simulink model "SHIP_DOWN_matlab_2017"  (R2018b)
settings: Solver=ode8  StartTime=0.0  StopTime=1  RelTol=1e-3
undefined symbols (not defined in the file): Cout_c, Cout_r, Cvh_c, Cvh_r, dellay_f1, dellay_f2, dellay_f3, dellay_f4, dellay_f5, dellay_f6, DiscIntNeverNeededParam, f, L1_l, L1_r, R_out, Uout, Uvh, Uvh_r
libraries: powerlib x40, simulink x7, simulink_extras x6, dspstat3 x4, powerlib_meascontrol x2
settings Model: Creator=Anton  LastModifiedBy=VID Company
settings SFSimCC: SimUseLocalCustomCode=off
settings RTWCC: RTWUseLocalCustomCode=off
settings CodeAppCC: StateflowObjectComments=on
settings SimscapeCC: SimscapeNormalizeSystem=off

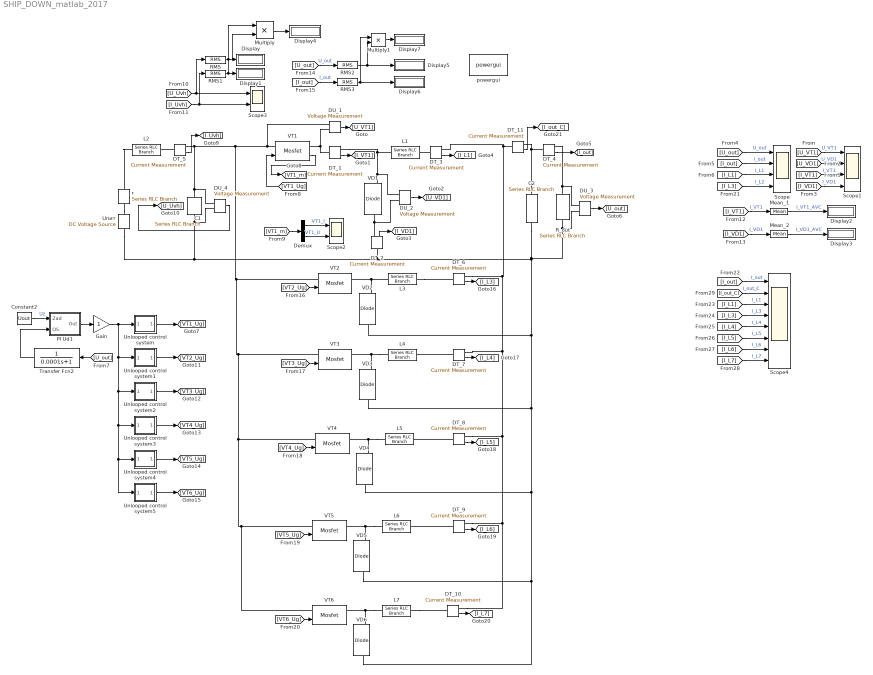
== system SHIP_DOWN_matlab_2017 ==
  C1 : powerlib/Elements/Series RLC Branch  LConnTagsString=__new0  RConnTagsString=__new0  BranchType=RC  Resistance=Cvh_r  Inductance=1e-3  SetiL0=off  InitialCurrent=0  Capacitance=Cvh_c  Setx0=on  InitialVoltage=Uvh  Measurements=Branch voltage
      settings: SourceProductName=Simscape Electrical
  C2 : powerlib/Elements/Series RLC Branch  LConnTagsString=__new0  RConnTagsString=__new0  BranchType=RC  Resistance=Cout_r  Inductance=1e-3  SetiL0=off  InitialCurrent=0  Capacitance=Cout_c  Setx0=on  InitialVoltage=Uout  Measurements=Branch voltage
      settings: SourceProductName=Simscape Electrical
  Constant2 : Constant  Value=Uout
  DT_{1..11} (11 alike) : powerlib/Measurements/Current Measurement  PhasorSimulation=off  OutputType=Complex  PSBequivalent=0
      settings: SourceProductName=Simscape Electrical
  DU_{1..4} (4 alike) : powerlib/Measurements/Voltage Measurement  PhasorSimulation=off  OutputType=Complex  PSBequivalent=0
      settings: SourceProductName=Simscape Electrical
  Demux : Demux  Outputs=2
  Display{,1..7} (8 alike) : Display
  Gain : Gain
  L{1,3..7} (6 alike) : powerlib/Elements/Series RLC Branch  LConnTagsString=__new0  RConnTagsString=__new0  BranchType=RL  Resistance=L1_r  Inductance=L1_l  SetiL0=off  InitialCurrent=0  Capacitance=1e-6  Setx0=off  InitialVoltage=0  Measurements=None
      settings: SourceProductName=Simscape Electrical
  L2 : powerlib/Elements/Series RLC Branch  LConnTagsString=__new0  RConnTagsString=__new0  BranchType=RL  Resistance=0  Inductance=L1_l/8  SetiL0=off  InitialCurrent=0  Capacitance=1e-6  Setx0=off  InitialVoltage=0  Measurements=None
      settings: SourceProductName=Simscape Electrical
  Mean_1 : powerlib_meascontrol/Measurements/Mean  Freq=5000  Vinit=0  Ts=0
  Mean_2 : powerlib_meascontrol/Measurements/Mean  Freq=5000  Vinit=0  Ts=0
  Multiply : Product
  Multiply1 : Product
  PI Ud1 : Subsystem
  RMS{,1..3} (4 alike) : dspstat3/RMS  run=off  directionMode=Each column  dimension=1  InputProcessing=Columns as channels (frame based)  reset_popup=None
  R_out : powerlib/Elements/Series RLC Branch  LConnTagsString=__new0  RConnTagsString=__new0  BranchType=R  Resistance=R_out  Inductance=1e-3  SetiL0=off  InitialCurrent=0  Capacitance=1e-6  Setx0=off  InitialVoltage=0  Measurements=None
      settings: SourceProductName=Simscape Electrical
  Scope : Scope  NumInputPorts=4
  Scope1 : Scope  NumInputPorts=4
  Scope2 : Scope  NumInputPorts=2
  Scope3 : Scope  NumInputPorts=2
  Scope4 : Scope  NumInputPorts=8
  Transfer Fcn2 : TransferFcn  Denominator=[0.0001 1]
  Unlooped control system : Subsystem
  Unlooped control system1 : Subsystem
  Unlooped control system2 : Subsystem
  Unlooped control system3 : Subsystem
  Unlooped control system4 : Subsystem
  Unlooped control system5 : Subsystem
  Uпит : powerlib/Electrical Sources/DC Voltage Source  Amplitude=Uvh  Measurements=None
      settings: SourceProductName=Simscape Electrical
  VD{1..6} (6 alike) : powerlib/Power Electronics/Diode  Ron=0.001  Lon=0  Vf=1  IC=0  UseSnubber=off  Rs=inf  Cs=inf  Measurements=on
      settings: SourceProductName=Simscape Electrical
  VT{1..6} (6 alike) : powerlib/Power Electronics/Mosfet  Ron=10e-3  Lon=inf  Rd=10e-3  Vfd=1  IC=0  Rs=1e5  Cs=inf  Measurements=on
      settings: SourceProductName=Simscape Electrical
  powergui : powerlib/powergui  Priority=1  SimulationMode=Discrete  SampleTime=1e-6  frequency=60  Iterations=50  frequencyindice=0  Pbase=100e6  ErrMax=1e-4  UnitsV=kV  UnitsW=MW  buscounter=0  FunctionMessages=off  echomessages=off  EnableUseOfTLC=off  CurrentSourceSwitches=off  DisableSnubberDevices=off  DisableRonSwitches=off  DisableVfSwitches=off  DisplayEquations=off  SolverType=Tustin/Backward Euler (TBE)  Interpol=off  ExternalGateDelay=off  methode=off  Ts=100  x0status=blocks  SPID=off  SwTol=0  HookPort=off  RestoreLinks=warning  ResistiveCurrentMeasurement=off  Frange=[0:2:500]  Ylog=off  Xlog=on  ShowGrid=off  save=off  variable=ZData  structure=0  ZoomFFT=off  StartTime=0.0  cycles=1  DisplayStyle=1  fundamental=60  FreqAxis=off  MaxFrequency=1000  frequencyindicesteady=1  RmsSteady=1  display=off
      settings: SourceProductName=Simscape Electrical
  r : powerlib/Elements/Series RLC Branch  LConnTagsString=__new0  RConnTagsString=__new0  BranchType=R  Resistance=Uvh_r  Inductance=1e-3  SetiL0=off  InitialCurrent=0  Capacitance=1e-6  Setx0=off  InitialVoltage=0  Measurements=None
      settings: SourceProductName=Simscape Electrical
  wires:
  Transfer Fcn2/1 -> PI Ud1/2(OS)
  PI Ud1/1(Out) -> Gain/1
  Constant2/1 -> PI Ud1/1(Zad)  "Uz"
  [U_VT1] -> Scope1/1  "U_VT1"
  DU_1/1 -> [U_VT1]
  DT_1/1 -> [I_VT1]
  [I_VT1] -> Scope1/3  "I_VT1"
  DU_2/1 -> [U_VD1]
  DT_2/1 -> [I_VD1]
  [I_VD1] -> Scope1/4  "I_VD1"
  [U_VD1] -> Scope1/2  "U_VD1"
  DT_3/1 -> [I_L1]
  DT_4/1 -> [I_out]
  DU_3/1 -> [U_out]
  [U_out] -> Scope/1  "U_out"
  [I_out] -> Scope/2  "I_out"
  [U_out] -> Transfer Fcn2/1
  [I_L1] -> Scope/3  "I_L1"
  [VT1_Ug] -> VT1/1
  Demux/1 -> Scope2/1  "VT1_I"
  Demux/2 -> Scope2/2  "VT1_U"
  VT1/1 -> [VT1_m]
  [VT1_m] -> Demux/1
  DT_5/1 -> [I_Uvh]
  DU_4/1 -> [U_Uvh]
  [I_Uvh] -> Scope3/2, RMS1/1
  [U_Uvh] -> Scope3/1, RMS/1
  RMS/1 -> Multiply/2, Display/1
  RMS1/1 -> Multiply/1, Display1/1
  Mean_1/1 -> Display2/1  "I_VT1_AVC"
  [I_VT1] -> Mean_1/1  "I_VT1"
  [I_VD1] -> Mean_2/1  "I_VD1"
  Mean_2/1 -> Display3/1  "I_VD1_AVC"
  Multiply/1 -> Display4/1
  [U_out] -> RMS2/1  "U_out"
  [I_out] -> RMS3/1  "I_out"
  Multiply1/1 -> Display7/1
  RMS2/1 -> Multiply1/2, Display5/1
  RMS3/1 -> Multiply1/1, Display6/1
  [VT2_Ug] -> VT2/1
  Unlooped control system/1(CH1) -> [VT1_Ug]
  Unlooped control system1/1(CH1) -> [VT2_Ug]
  [VT3_Ug] -> VT3/1
  [VT4_Ug] -> VT4/1
  [VT5_Ug] -> VT5/1
  [VT6_Ug] -> VT6/1
  Gain/1 -> Unlooped control system/1(Uz), Unlooped control system5/1(Uz), Unlooped control system4/1(Uz), Unlooped control system3/1(Uz), Unlooped control system2/1(Uz), Unlooped control system1/1(Uz)
  Unlooped control system2/1(CH1) -> [VT3_Ug]
  Unlooped control system3/1(CH1) -> [VT4_Ug]
  Unlooped control system4/1(CH1) -> [VT5_Ug]
  Unlooped control system5/1(CH1) -> [VT6_Ug]
  DT_6/1 -> [I_L3]
  [I_L3] -> Scope/4  "I_L2"
  DT_7/1 -> [I_L4]
  DT_8/1 -> [I_L5]
  DT_9/1 -> [I_L6]
  DT_10/1 -> [I_L7]
  [I_out] -> Scope4/1  "I_out"
  DT_11/1 -> [I_out_C]
  [I_L1] -> Scope4/3  "I_L1"
  [I_L3] -> Scope4/4  "I_L3"
  [I_L4] -> Scope4/5  "I_L4"
  [I_L5] -> Scope4/6  "I_L5"
  [I_L6] -> Scope4/7  "I_L6"
  [I_L7] -> Scope4/8  "I_L7"
  [I_out_C] -> Scope4/2  "I_out_C"
  connections:
  C1/RConn1 -- DT_2/LConn1 -- DU_3/LConn2 -- R_out/RConn1 -- C2/RConn1 -- VD6/LConn1 -- VD5/LConn1 -- VD4/LConn1 -- VD3/LConn1 -- VD2/LConn1 -- Uпит/LConn1 -- DU_4/LConn2
  r/RConn1 -- Uпит/RConn1
  DT_4/RConn1 -- DU_3/LConn1 -- R_out/LConn1
  L1/LConn1 -- DT_1/RConn1 -- DU_2/LConn1 -- VD1/RConn1
  DT_3/LConn1 -- L1/RConn1
  VD1/LConn1 -- DT_2/RConn1 -- DU_2/LConn2
  DU_1/LConn2 -- DT_1/LConn1 -- VT1/RConn1
  DU_4/LConn1 -- VT6/LConn1 -- VT5/LConn1 -- VT4/LConn1 -- VT3/LConn1 -- VT2/LConn1 -- DU_1/LConn1 -- VT1/LConn1 -- DT_5/RConn1 -- C1/LConn1
  DT_5/LConn1 -- L2/RConn1
  L2/LConn1 -- r/LConn1
  VD2/RConn1 -- VT2/RConn1 -- L3/LConn1
  L4/LConn1 -- VT3/RConn1 -- VD3/RConn1
  L5/LConn1 -- VT4/RConn1 -- VD4/RConn1
  L6/LConn1 -- VT5/RConn1 -- VD5/RConn1
  L7/LConn1 -- VT6/RConn1 -- VD6/RConn1
  DT_6/RConn1 -- DT_10/RConn1 -- DT_9/RConn1 -- DT_8/RConn1 -- DT_7/RConn1 -- DT_11/LConn1 -- DT_3/RConn1
  L3/RConn1 -- DT_6/LConn1
  DT_7/LConn1 -- L4/RConn1
  DT_8/LConn1 -- L5/RConn1
  DT_9/LConn1 -- L6/RConn1
  L7/RConn1 -- DT_10/LConn1
  C2/LConn1 -- DT_11/RConn1 -- DT_4/LConn1

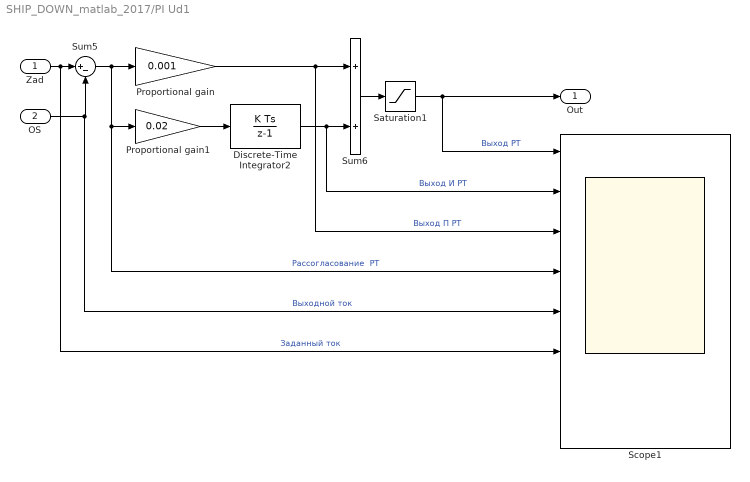
== system SHIP_DOWN_matlab_2017/PI Ud1 ==
  Zad : Inport
  OS : Inport  Port=2
  Discrete-Time Integrator2 : DiscreteIntegrator  SampleTime=-1  LimitOutput=on  UpperSaturationLimit=0.9  LowerSaturationLimit=0  ICPrevOutput=DiscIntNeverNeededParam  ICPrevScaledInput=DiscIntNeverNeededParam
  Proportional gain : Gain  Gain=0.001  SaturateOnIntegerOverflow=on  OutDataTypeStr=Inherit: Same as input  ParamDataTypeStr=Inherit: Same as input
  Proportional gain1 : Gain  Gain=0.02  SaturateOnIntegerOverflow=on  OutDataTypeStr=Inherit: Same as input  ParamDataTypeStr=Inherit: Same as input
  Saturation1 : Saturate  UpperLimit=0.9  LowerLimit=0
  Scope1 : Scope  NumInputPorts=8
  Sum5 : Sum  Inputs=|+-  SaturateOnIntegerOverflow=on  InputSameDT=on  OutDataTypeStr=Inherit: Same as first input
  Sum6 : Sum  SaturateOnIntegerOverflow=on  InputSameDT=on  OutDataTypeStr=Inherit: Same as first input
  Out : Outport
  wires:
  Proportional gain/1 -> Scope1/3, Sum6/1  "Выход П РТ"
  Discrete-Time Integrator2/1 -> Sum6/2, Scope1/2  "Выход И РТ"
  OS/1 -> Scope1/5, Sum5/2  "Выходной ток"
  Zad/1 -> Scope1/6, Sum5/1  "Заданный ток"
  Sum5/1 -> Proportional gain1/1, Scope1/4, Proportional gain/1  "Рассогласование  РТ"
  Sum6/1 -> Saturation1/1
  Saturation1/1 -> Out/1, Scope1/1  "Выход РТ"
  Proportional gain1/1 -> Discrete-Time Integrator2/1

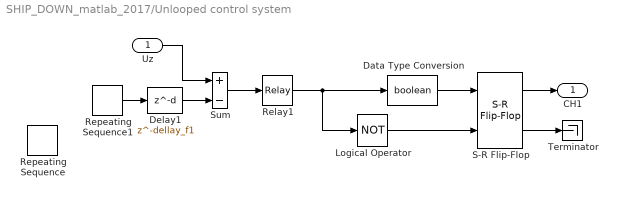
== system SHIP_DOWN_matlab_2017/Unlooped control system ==
  Uz : Inport
  Data Type Conversion : DataTypeConversion  OutDataTypeStr=boolean
  Delay1 : Delay  DelayLength=dellay_f1  InitialCondition=0  UseCircularBuffer=on
  Logical Operator : Logic  Operator=NOT  AllPortsSameDT=off  OutDataTypeStr=boolean
  Relay1 : Relay  OnSwitchValue=0.01  OffSwitchValue=-0.01
  Repeating Sequence : simulink/Sources/Repeating Sequence  rep_seq_t=[0 0.00025]  rep_seq_y=[0 1]
  Repeating Sequence1 : simulink/Sources/Repeating Sequence  rep_seq_t="[0  (1/(2*f)) (1/f)]"  rep_seq_y=[0 1 0]
  S-R Flip-Flop : simulink_extras/Flip Flops/S-R Flip-Flop  initial_condition=0
  Sum : Sum  Inputs=+-
  Terminator : Terminator
  CH1 : Outport
  wires:
  S-R Flip-Flop/1 -> CH1/1
  Data Type Conversion/1 -> S-R Flip-Flop/1
  Logical Operator/1 -> S-R Flip-Flop/2
  Relay1/1 -> Logical Operator/1, Data Type Conversion/1
  Uz/1 -> Sum/1
  Sum/1 -> Relay1/1
  S-R Flip-Flop/2 -> Terminator/1
  Repeating Sequence1/1 -> Delay1/1
  Delay1/1 -> Sum/2

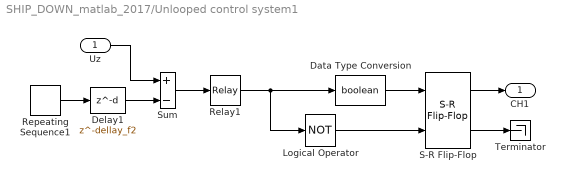
== system SHIP_DOWN_matlab_2017/Unlooped control system1 ==
  Uz : Inport
  Data Type Conversion : DataTypeConversion  OutDataTypeStr=boolean
  Delay1 : Delay  DelayLength=dellay_f2  InitialCondition=0  UseCircularBuffer=on
  Logical Operator : Logic  Operator=NOT  AllPortsSameDT=off  OutDataTypeStr=boolean
  Relay1 : Relay  OnSwitchValue=0.01  OffSwitchValue=-0.01
  Repeating Sequence1 : simulink/Sources/Repeating Sequence  rep_seq_t="[0  (1/(2*f)) (1/f)]"  rep_seq_y=[0 1 0]
  S-R Flip-Flop : simulink_extras/Flip Flops/S-R Flip-Flop  initial_condition=0
  Sum : Sum  Inputs=+-
  Terminator : Terminator
  CH1 : Outport
  wires:
  S-R Flip-Flop/1 -> CH1/1
  Data Type Conversion/1 -> S-R Flip-Flop/1
  Logical Operator/1 -> S-R Flip-Flop/2
  Relay1/1 -> Logical Operator/1, Data Type Conversion/1
  Uz/1 -> Sum/1
  Sum/1 -> Relay1/1
  S-R Flip-Flop/2 -> Terminator/1
  Repeating Sequence1/1 -> Delay1/1
  Delay1/1 -> Sum/2

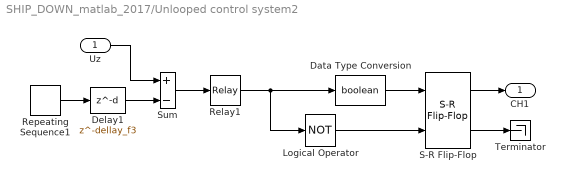
== system SHIP_DOWN_matlab_2017/Unlooped control system2 ==
  Uz : Inport
  Data Type Conversion : DataTypeConversion  OutDataTypeStr=boolean
  Delay1 : Delay  DelayLength=dellay_f3  InitialCondition=0  UseCircularBuffer=on
  Logical Operator : Logic  Operator=NOT  AllPortsSameDT=off  OutDataTypeStr=boolean
  Relay1 : Relay  OnSwitchValue=0.01  OffSwitchValue=-0.01
  Repeating Sequence1 : simulink/Sources/Repeating Sequence  rep_seq_t="[0  (1/(2*f)) (1/f)]"  rep_seq_y=[0 1 0]
  S-R Flip-Flop : simulink_extras/Flip Flops/S-R Flip-Flop  initial_condition=0
  Sum : Sum  Inputs=+-
  Terminator : Terminator
  CH1 : Outport
  wires:
  S-R Flip-Flop/1 -> CH1/1
  Data Type Conversion/1 -> S-R Flip-Flop/1
  Logical Operator/1 -> S-R Flip-Flop/2
  Relay1/1 -> Logical Operator/1, Data Type Conversion/1
  Uz/1 -> Sum/1
  Sum/1 -> Relay1/1
  S-R Flip-Flop/2 -> Terminator/1
  Repeating Sequence1/1 -> Delay1/1
  Delay1/1 -> Sum/2

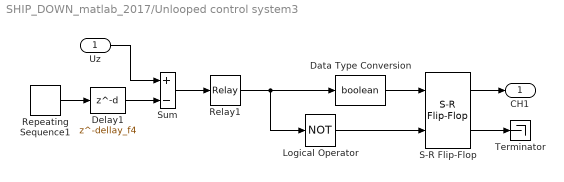
== system SHIP_DOWN_matlab_2017/Unlooped control system3 ==
  Uz : Inport
  Data Type Conversion : DataTypeConversion  OutDataTypeStr=boolean
  Delay1 : Delay  DelayLength=dellay_f4  InitialCondition=0  UseCircularBuffer=on
  Logical Operator : Logic  Operator=NOT  AllPortsSameDT=off  OutDataTypeStr=boolean
  Relay1 : Relay  OnSwitchValue=0.01  OffSwitchValue=-0.01
  Repeating Sequence1 : simulink/Sources/Repeating Sequence  rep_seq_t="[0  (1/(2*f)) (1/f)]"  rep_seq_y=[0 1 0]
  S-R Flip-Flop : simulink_extras/Flip Flops/S-R Flip-Flop  initial_condition=0
  Sum : Sum  Inputs=+-
  Terminator : Terminator
  CH1 : Outport
  wires:
  S-R Flip-Flop/1 -> CH1/1
  Data Type Conversion/1 -> S-R Flip-Flop/1
  Logical Operator/1 -> S-R Flip-Flop/2
  Relay1/1 -> Logical Operator/1, Data Type Conversion/1
  Uz/1 -> Sum/1
  Sum/1 -> Relay1/1
  S-R Flip-Flop/2 -> Terminator/1
  Repeating Sequence1/1 -> Delay1/1
  Delay1/1 -> Sum/2

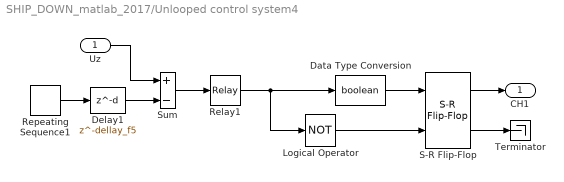
== system SHIP_DOWN_matlab_2017/Unlooped control system4 ==
  Uz : Inport
  Data Type Conversion : DataTypeConversion  OutDataTypeStr=boolean
  Delay1 : Delay  DelayLength=dellay_f5  InitialCondition=0  UseCircularBuffer=on
  Logical Operator : Logic  Operator=NOT  AllPortsSameDT=off  OutDataTypeStr=boolean
  Relay1 : Relay  OnSwitchValue=0.01  OffSwitchValue=-0.01
  Repeating Sequence1 : simulink/Sources/Repeating Sequence  rep_seq_t="[0  (1/(2*f)) (1/f)]"  rep_seq_y=[0 1 0]
  S-R Flip-Flop : simulink_extras/Flip Flops/S-R Flip-Flop  initial_condition=0
  Sum : Sum  Inputs=+-
  Terminator : Terminator
  CH1 : Outport
  wires:
  S-R Flip-Flop/1 -> CH1/1
  Data Type Conversion/1 -> S-R Flip-Flop/1
  Logical Operator/1 -> S-R Flip-Flop/2
  Relay1/1 -> Logical Operator/1, Data Type Conversion/1
  Uz/1 -> Sum/1
  Sum/1 -> Relay1/1
  S-R Flip-Flop/2 -> Terminator/1
  Repeating Sequence1/1 -> Delay1/1
  Delay1/1 -> Sum/2

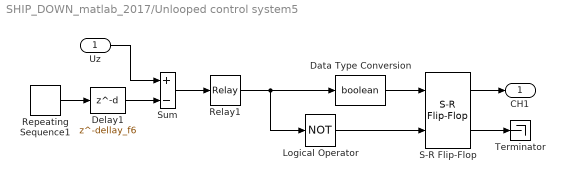
== system SHIP_DOWN_matlab_2017/Unlooped control system5 ==
  Uz : Inport
  Data Type Conversion : DataTypeConversion  OutDataTypeStr=boolean
  Delay1 : Delay  DelayLength=dellay_f6  InitialCondition=0  UseCircularBuffer=on
  Logical Operator : Logic  Operator=NOT  AllPortsSameDT=off  OutDataTypeStr=boolean
  Relay1 : Relay  OnSwitchValue=0.01  OffSwitchValue=-0.01
  Repeating Sequence1 : simulink/Sources/Repeating Sequence  rep_seq_t="[0  (1/(2*f)) (1/f)]"  rep_seq_y=[0 1 0]
  S-R Flip-Flop : simulink_extras/Flip Flops/S-R Flip-Flop  initial_condition=0
  Sum : Sum  Inputs=+-
  Terminator : Terminator
  CH1 : Outport
  wires:
  S-R Flip-Flop/1 -> CH1/1
  Data Type Conversion/1 -> S-R Flip-Flop/1
  Logical Operator/1 -> S-R Flip-Flop/2
  Relay1/1 -> Logical Operator/1, Data Type Conversion/1
  Uz/1 -> Sum/1
  Sum/1 -> Relay1/1
  S-R Flip-Flop/2 -> Terminator/1
  Repeating Sequence1/1 -> Delay1/1
  Delay1/1 -> Sum/2
